simulink subsystem "ControlObject"  (R2025a)
settings: Solver=VariableStepAuto  StartTime=0.0  StopTime=10.0  RelTol=1e-3
settings Model: Creator=Глеб  LastModifiedBy=Глеб

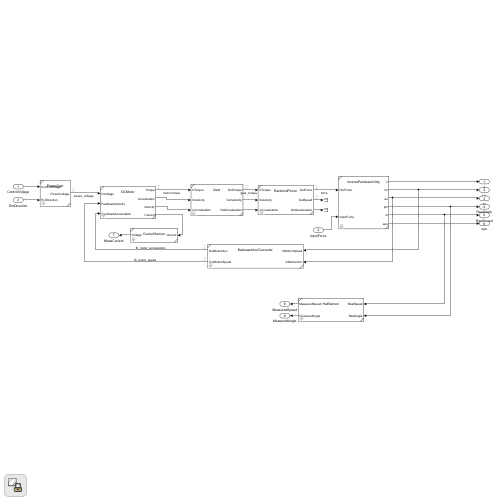
[thumbnail: Simulink's stored preview of the top-level diagram]
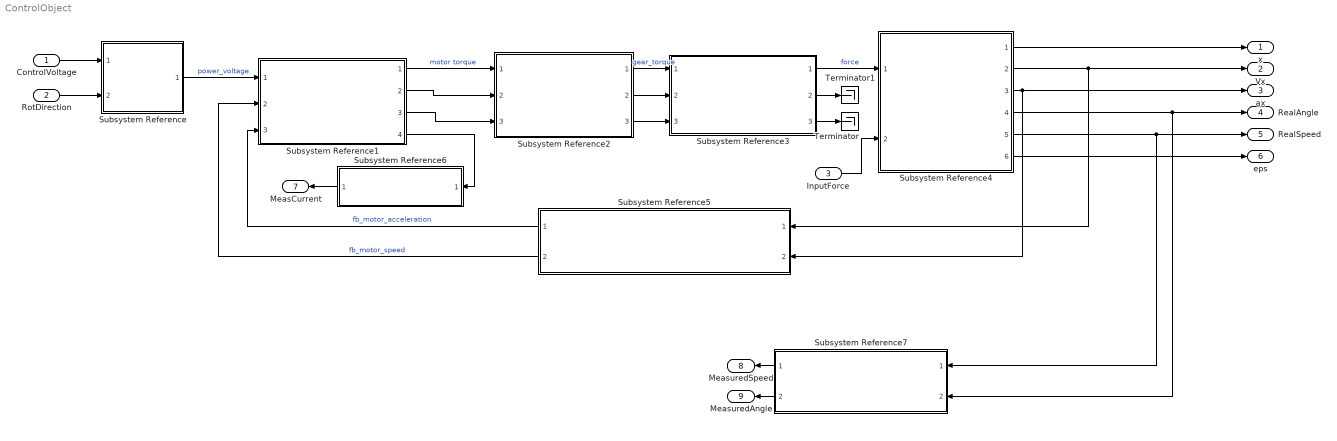
== system ControlObject ==
  ControlVoltage : Inport
  RotDirection : Inport  Port=2
  InputForce : Inport  Port=3
  Subsystem Reference : Subsystem  ReferencedSubsystem=PowerGain  gain=24/3.3
  Subsystem Reference1 : Subsystem  ReferencedSubsystem=DCMotor  kw=1/60  L=350*10^-6  R=10  km=16/1000  J_motor=500*10^-9  vis_friction_coef_motor=0.001
  Subsystem Reference2 : Subsystem  ReferencedSubsystem=Gear  i_gear=100  J_gear=2.4*10^-6  vis_friction_coef_gear=0.001
  Subsystem Reference3 : Subsystem  ReferencedSubsystem=RackAndPinion  i_coef=20/1000  J_pinion=1*10^-6  m_rack=0.1  vis_friction_coef_rack=0.001
  Subsystem Reference4 : Subsystem  ReferencedSubsystem=InversePendulumOnly  m_p=0.2  m_c=0.1  l_c=0.5  g=9.81  J_p=0.0667  phi0=0.087
  Subsystem Reference5 : Subsystem  ReferencedSubsystem=BackwardAccConverter  k_rack=20  i_gear=100
  Subsystem Reference6 : Subsystem  ReferencedSubsystem=CurrentSensor  R=0.001
  Subsystem Reference7 : Subsystem  ReferencedSubsystem=HallSensor  kw=0.2  kphi=2
  Terminator : Terminator
  Terminator1 : Terminator
  x : Outport
  Vx : Outport  Port=2
  ax : Outport  Port=3
  RealAngle : Outport  Port=4
  RealSpeed : Outport  Port=5
  eps : Outport  Port=6
  MeasCurrent : Outport  Port=7
  MeasuredSpeed : Outport  Port=8
  MeasuredAngle : Outport  Port=9
  wires:
  Subsystem Reference7/1 -> MeasuredSpeed/1
  ControlVoltage/1 -> Subsystem Reference/1
  Subsystem Reference3/3 -> Terminator/1
  RotDirection/1 -> Subsystem Reference/2
  Subsystem Reference/1 -> Subsystem Reference1/1  "power_voltage"
  Subsystem Reference4/3 -> Subsystem Reference5/2, ax/1
  Subsystem Reference1/3 -> Subsystem Reference2/3
  Subsystem Reference4/5 -> RealSpeed/1, Subsystem Reference7/1
  Subsystem Reference2/3 -> Subsystem Reference3/3
  Subsystem Reference1/1 -> Subsystem Reference2/1  "motor torque"
  Subsystem Reference6/1 -> MeasCurrent/1
  Subsystem Reference2/1 -> Subsystem Reference3/1  "gear_torque"
  Subsystem Reference7/2 -> MeasuredAngle/1
  Subsystem Reference5/2 -> Subsystem Reference1/2  "fb_motor_speed"
  InputForce/1 -> Subsystem Reference4/2
  Subsystem Reference1/4 -> Subsystem Reference6/1
  Subsystem Reference4/6 -> eps/1
  Subsystem Reference3/2 -> Terminator1/1
  Subsystem Reference2/2 -> Subsystem Reference3/2
  Subsystem Reference1/2 -> Subsystem Reference2/2
  Subsystem Reference5/1 -> Subsystem Reference1/3  "fb_motor_acceleration"
  Subsystem Reference4/1 -> x/1
  Subsystem Reference4/2 -> Subsystem Reference5/1, Vx/1
  Subsystem Reference4/4 -> RealAngle/1, Subsystem Reference7/2
  Subsystem Reference3/1 -> Subsystem Reference4/1  "force"
